simulink model "fest_komma2"  (Simulink 7.8)
settings: Solver=ode45  StartTime=0.0  StopTime=10.0  RelTol=1e-3
libraries: simulink x1
settings Model: Creator=svenhoffmann  LastModifiedBy=josef  ExtModeAutoUpdateStatusClock=off
settings DataIOCC: TimeSaveName=t  OutputSaveName=y  SignalLoggingName=sigsOut
settings OptimizationCC: InlineInvariantSignals=on  InitFltsAndDblsToZero=on
settings DebuggingCC: SaveWithParameterizedLinksMsg=none  SignalResolutionControl=TryResolveAllWithWarning  SolverPrmCheckMsg=none  MultiTaskDSMMsg=warning  MultiTaskCondExecSysMsg=none  FcnCallInpInsideContextMsg=Use local settings  StrictBusMsg=None
settings HardwareCC: TargetUnknown=on
settings RTWCC: IncludeERTFirstTime=on
settings GRTTargetCC: TargetFcnLib=ansi_tfl_tmw.mat

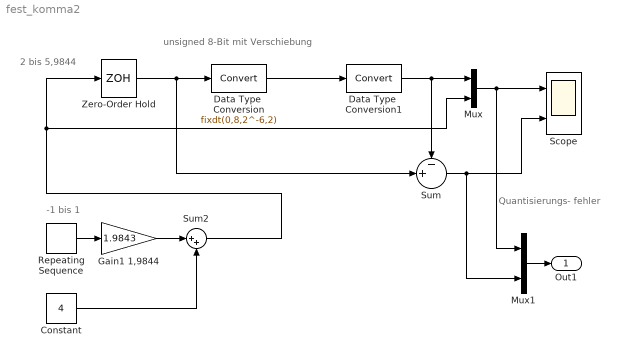
== system fest_komma2 ==
  note: -1 bis 1
  note: unsigned 8-Bit
      | mit Verschiebung
  note: Quantisierungs-
      | fehler
  note: 2 bis 5,9844
  Constant : Constant  Value=4
  Data Type  Conversion : DataTypeConversion  OutDataTypeStr=fixdt(0,8,2^-6,2)  RndMeth=Nearest  SaturateOnIntegerOverflow=on
  Data Type  Conversion1 : DataTypeConversion  RndMeth=Nearest  SaturateOnIntegerOverflow=on
  Gain1 1,9844 : Gain  Gain=1.9843  SaturateOnIntegerOverflow=on  OutDataTypeStr=Inherit: Same as input  ParamDataTypeStr=Inherit: Same as input
  Mux : Mux  Inputs=2
  Mux1 : Mux  Inputs=2
  Repeating Sequence : simulink/Sources/Repeating Sequence  rep_seq_t=[0 1 2]  rep_seq_y=[-1 1 -1]
  Scope : Scope  NumInputPorts=2
      settings: YMin=-5~-5  YMax=5~5
  Sum : Sum  Inputs=-+|  SaturateOnIntegerOverflow=on  InputSameDT=on  OutDataTypeStr=Inherit: Same as first input
  Sum2 : Sum  Inputs=|++  SaturateOnIntegerOverflow=on  InputSameDT=on  OutDataTypeStr=Inherit: Same as first input
  Zero-Order Hold : ZeroOrderHold  SampleTime=1/100
  Out1 : Outport
  wires:
  Zero-Order Hold/1 -> Sum/2, Data Type  Conversion/1
  Data Type  Conversion/1 -> Data Type  Conversion1/1
  Data Type  Conversion1/1 -> Mux/1, Sum/1
  Mux/1 -> Scope/1, Mux1/1
  Sum/1 -> Scope/2, Mux1/2
  Repeating Sequence/1 -> Gain1 1,9844/1
  Gain1 1,9844/1 -> Sum2/1
  Constant/1 -> Sum2/2
  Mux1/1 -> Out1/1
  Sum2/1 -> Zero-Order Hold/1, Mux/2
